simulink model "THEFINAL"  (R2020b)
settings: Solver=VariableStepAuto  StartTime=0.0  StopTime=60  RelTol=1e-3
values from neighbouring files (symbols this model uses):
  A_2 = zeros(3)    [Trial_Script.m]
  A_AD = horzcat(A_i, A_ii)    [Trial_Script.m]
  A_kal = [0 0 0 1 0 0 ... (first row only)    [Trial_Script.m]
  B_2 = I_inv    [Trial_Script.m]
  B_AD = horzcat(B_i, B_ii)    [Trial_Script.m]
  B_kal = [0 0 0 0 0 0 ... (first row only)    [Trial_Script.m]
  C_2 = eye(3)    [Trial_Script.m]
  C_AD = eye(6)    [Trial_Script.m]
  C_kal = eye(6)    [Trial_Script.m]
  D_2 = zeros(3)    [Trial_Script.m]
  D_AD = zeros(6)    [Trial_Script.m]
  D_kal = zeros(6)    [Trial_Script.m]
  f_prop = 100    [Trial_Script.m]
  Fb1_l = -100000    [Trial_Script.m]
  Fb1_u = 100000    [Trial_Script.m]
  Fb2_l = -100000    [Trial_Script.m]
  Fb2_u = 100000    [Trial_Script.m]
  Fb3_l = -100000    [Trial_Script.m]
  Fb3_u = 100000    [Trial_Script.m]
  Fb4_l = -100000    [Trial_Script.m]
  Fb4_u = 100000    [Trial_Script.m]
  Fc1_l = -30000    [Trial_Script.m]
  Fc1_u = 30000    [Trial_Script.m]
  Fc2_l = -30000    [Trial_Script.m]
  Fc2_u = 30000    [Trial_Script.m]
  Fc3_l = -30000    [Trial_Script.m]
  Fc3_u = 30000    [Trial_Script.m]
  Ft1_l = -100000    [Trial_Script.m]
  Ft1_u = 100000    [Trial_Script.m]
  Ft2_l = -100000    [Trial_Script.m]
  Ft2_u = 100000    [Trial_Script.m]
  Ft3_l = -100000    [Trial_Script.m]
  Ft3_u = 100000    [Trial_Script.m]
  Ft4_l = -100000    [Trial_Script.m]
  Ft4_u = 100000    [Trial_Script.m]
  g = 9.81    [Trial_Script.m]
  m = 645    [Trial_Script.m]    (also in testing_file.m = (abs(max(z)) + abs(min(z)))/(abs(max(y)) + abs(min(y))); wind_stuff.m = (abs(max(z)) + abs(min(z)))/(abs(max(y)) + abs(min(y))))
  r_0 = Tzy_Shard*[90; -125; 160]    [Trial_Script.m]
  rho = 1.225    [Trial_Script.m]
  T = 10.5    [Trial_Script.m]
  time_delay = 0.1    [Trial_Script.m]
  Tx_aero = [1 0 0 ... (first row only)    [Trial_Script.m]
  Tzy_Shard = [cos(pi/2) -sin(pi/2) 0; sin(pi/2) cos(pi/2) 0; 0 0 1]*[1 0 0 ... (first row only)    [Reading_Shard_Data.m]    (also in Trial_Script.m)
  Tzy_Shard_inv = inv(Tzy_Shard)    [Trial_Script.m]
  u_0 = a(1:d,1)    [Reading_Shard_Data.m]    (also in Trial_Script.m = a(1:d_shard,1); testing_file.m)
  u_1 = a(1:d,2)    [Reading_Shard_Data.m]    (also in Trial_Script.m = a(1:d_shard,2); testing_file.m)
  u_2 = a(1:d,3)    [Reading_Shard_Data.m]    (also in Trial_Script.m = a(1:d_shard,3); testing_file.m)
  v_0 = Tzy_Shard*V0_shard    [Trial_Script.m]
  w_0 = [0;0;0]    [Trial_Script.m]
  xdata = a(1:d_shard,4)    [Trial_Script.m]
  ydata = a(1:d_shard,5)    [Trial_Script.m]
  zdata = a(1:d_shard,6)    [Trial_Script.m]
  ZI_Cx = model_Cx(XI_Cx, YI_Cx)    [Trial_Script.m]
  ZI_Cy = model_Cy(XI_Cy, YI_Cy)    [Trial_Script.m]
  ZI_Cz = model_Cz(XI_Cz, YI_Cz)    [Trial_Script.m]
  ZI_p = model_p(XI_p, YI_p)    [Trial_Script.m]
  ZI_q = model_q(XI_q, YI_q)    [Trial_Script.m]
  ZI_r = model_r(XI_r, YI_r)    [Trial_Script.m]
undefined symbols (not defined in the file or in its folder): C_D, Continuous, S, Time
libraries: pid_lib x3, dspsigops x3, fuzblock x3, dspindex x3, ctrlSharedLib x2, simulink x1, mpclib x1, dspmathops x1, cstblocks x1
(part 2 of 2)

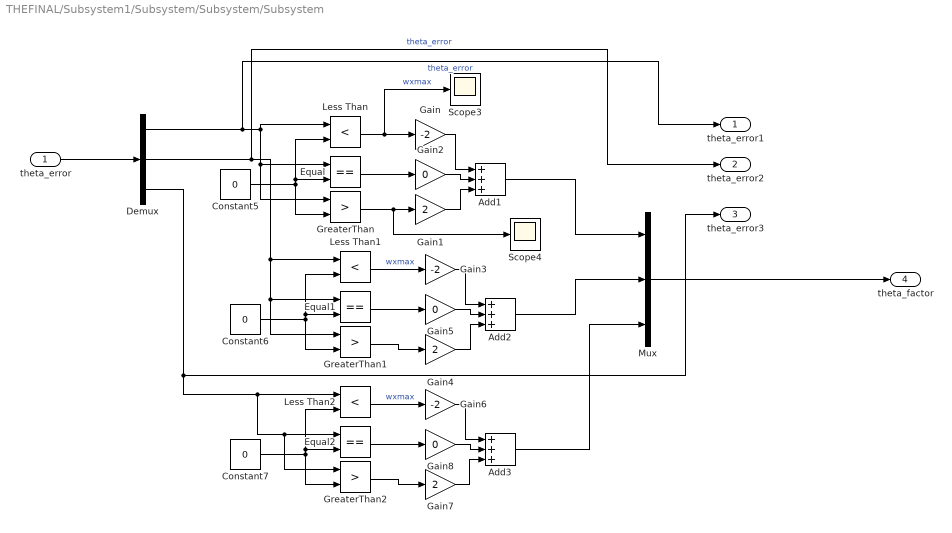
== system THEFINAL/Subsystem1/Subsystem/Subsystem/Subsystem ==
  theta_error : Inport
  Add1 : Sum  Inputs=+++
  Add2 : Sum  Inputs=+++
  Add3 : Sum  Inputs=+++
  Constant5 : Constant  Value=0
  Constant6 : Constant  Value=0
  Constant7 : Constant  Value=0
  Demux : Demux  Outputs=3
  Equal : RelationalOperator  Operator===  OutDataTypeStr=boolean  RndMeth=Simplest
  Equal1 : RelationalOperator  Operator===  OutDataTypeStr=boolean  RndMeth=Simplest
  Equal2 : RelationalOperator  Operator===  OutDataTypeStr=boolean  RndMeth=Simplest
  Gain : Gain  Gain=-2
  Gain1 : Gain  Gain=2
  Gain2 : Gain  Gain=0
  Gain3 : Gain  Gain=-2
  Gain4 : Gain  Gain=2
  Gain5 : Gain  Gain=0
  Gain6 : Gain  Gain=-2
  Gain7 : Gain  Gain=2
  Gain8 : Gain  Gain=0
  GreaterThan : RelationalOperator  Operator=>  OutDataTypeStr=boolean  RndMeth=Simplest
  GreaterThan1 : RelationalOperator  Operator=>  OutDataTypeStr=boolean  RndMeth=Simplest
  GreaterThan2 : RelationalOperator  Operator=>  OutDataTypeStr=boolean  RndMeth=Simplest
  Less Than : RelationalOperator  Operator=<  OutDataTypeStr=boolean  RndMeth=Simplest
  Less Than1 : RelationalOperator  Operator=<  OutDataTypeStr=boolean  RndMeth=Simplest
  Less Than2 : RelationalOperator  Operator=<  OutDataTypeStr=boolean  RndMeth=Simplest
  Mux : Mux  Inputs=3
  Scope3 : Scope
  Scope4 : Scope
  theta_error1 : Outport
  theta_error2 : Outport  Port=2
  theta_error3 : Outport  Port=3
  theta_factor : Outport  Port=4
  wires:
  Add1/1 -> Mux/1
  Constant5/1 -> Equal/2, Less Than/2, GreaterThan/2
  Equal2/1 -> Gain8/1
  Demux/1 -> theta_error1/1, GreaterThan/1, Equal/1, Less Than/1  "theta_error"
  GreaterThan2/1 -> Gain7/1
  Gain1/1 -> Add1/3
  Gain7/1 -> Add3/3
  Less Than1/1 -> Gain3/1  "wxmax"
  Gain6/1 -> Add3/1
  Equal/1 -> Gain2/1
  Gain5/1 -> Add2/2
  Add3/1 -> Mux/3
  GreaterThan/1 -> Scope4/1, Gain1/1
  Constant6/1 -> Equal1/2, Less Than1/2, GreaterThan1/2
  Demux/3 -> theta_error3/1, GreaterThan2/1, Equal2/1, Less Than2/1
  Gain3/1 -> Add2/1
  Constant7/1 -> Equal2/2, Less Than2/2, GreaterThan2/2
  Equal1/1 -> Gain5/1
  Gain8/1 -> Add3/2
  Gain4/1 -> Add2/3
  GreaterThan1/1 -> Gain4/1
  Gain/1 -> Add1/1
  Demux/2 -> theta_error2/1, GreaterThan1/1, Equal1/1, Less Than1/1  "theta_error"
  Gain2/1 -> Add1/2
  Add2/1 -> Mux/2
  Less Than/1 -> Scope3/1, Gain/1  "wxmax"
  Less Than2/1 -> Gain6/1  "wxmax"
  theta_error/1 -> Demux/1
  Mux/1 -> theta_factor/1

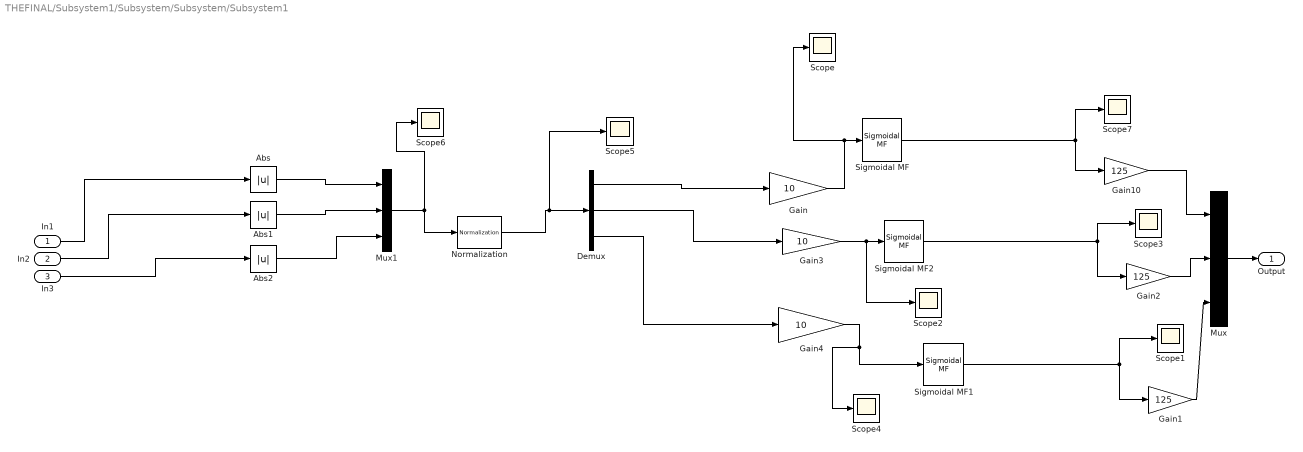
== system THEFINAL/Subsystem1/Subsystem/Subsystem/Subsystem1 ==
  In1 : Inport
  In2 : Inport  Port=2
  In3 : Inport  Port=3
  Abs : Abs
  Abs1 : Abs
  Abs2 : Abs
  Demux : Demux  Outputs=3
  Gain : Gain  Gain=10
  Gain1 : Gain  Gain=125
  Gain10 : Gain  Gain=125
  Gain2 : Gain  Gain=125
  Gain3 : Gain  Gain=10
  Gain4 : Gain  Gain=10
  Mux : Mux  Inputs=3
  Mux1 : Mux  Inputs=3
  Normalization : dspmathops/Normalization  NormType=Squared 2-norm  Bias=1e-10  NormOver=Each column  Dimension=1  roundingMode=Floor  overflowMode=off  accumDataTypeStr=Inherit: Same as product output  accumLastDataTypeStr=Inherit: Same as product output  outputDataTypeStr=Inherit: Same as product output  outputMin=[]  outputMax=[]  outputLastDataTypeStr=Inherit: Same as product output
  Scope{,1..7} (8 alike) : Scope
  Sigmoidal MF : fuzblock/Membership  Functions/Sigmoidal MF  a=10^(-8)  c=1000
      settings: SourceProductBaseCode=FL
  Sigmoidal MF1 : fuzblock/Membership  Functions/Sigmoidal MF  a=10^(-8)  c=1000
      settings: SourceProductBaseCode=FL
  Sigmoidal MF2 : fuzblock/Membership  Functions/Sigmoidal MF  a=10^(-8)  c=1000
      settings: SourceProductBaseCode=FL
  Output : Outport
  wires:
  Gain2/1 -> Mux/2
  Gain10/1 -> Mux/1
  Sigmoidal MF1/1 -> Gain1/1, Scope1/1
  Sigmoidal MF/1 -> Gain10/1, Scope7/1
  Sigmoidal MF2/1 -> Gain2/1, Scope3/1
  Gain/1 -> Scope/1, Sigmoidal MF/1
  Gain1/1 -> Mux/3
  Gain3/1 -> Scope2/1, Sigmoidal MF2/1
  In2/1 -> Abs1/1
  In1/1 -> Abs/1
  In3/1 -> Abs2/1
  Mux/1 -> Output/1
  Abs/1 -> Mux1/1
  Abs1/1 -> Mux1/2
  Gain4/1 -> Scope4/1, Sigmoidal MF1/1
  Abs2/1 -> Mux1/3
  Demux/3 -> Gain4/1
  Demux/1 -> Gain/1
  Demux/2 -> Gain3/1
  Mux1/1 -> Normalization/1, Scope6/1
  Normalization/1 -> Scope5/1, Demux/1

== matlab function THEFINAL/Transformation Subsystem/MATLAB Function2 ==
  data: theta_x input; Transformation_Mat output; theta_y input; theta_z input
function Transformation_Mat  = Euler(theta_x, theta_y, theta_z)

a = cos(theta_x)*cos(theta_z);
b = cos(theta_x)*sin(theta_z);
c = - sin(theta_x);
d = sin(theta_y)*sin(theta_x)*cos(theta_z) - cos(theta_y)*sin(theta_z);
e = sin(theta_y)*sin(theta_x)*sin(theta_z) + cos(theta_y)*cos(theta_z);
f = sin(theta_y)*cos(theta_x);
g = cos(theta_y)*sin(theta_x)*cos(theta_z) + sin(theta_y)*sin(theta_z);
h = cos(theta_y)*sin(theta_x)*sin(theta_z) - sin(theta_y)*cos(theta_z);
i = cos(theta_y)*cos(theta_x);

Transformation_Mat = [a b c;
    d e f;
    g h i];


end

== matlab function THEFINAL/GPS model/GPS Model ==
  settings: updateMethod=DISCRETE
  data: position input; newposition output
function newposition  = gps(position)

    % Input: position
    % Output: position with gps accuracies inclduded
    mu = 0; 
    sigma = 0.015;

    r1 = normrnd(mu, sigma);
    r2 = normrnd(mu, sigma);
    r3 = normrnd(mu, sigma);

    newposition = [0,0,0];

    newposition(1) = position(1) + r1;
    newposition(2) = position(2) + r2;
    newposition(3) = position(3) + r3;

end

== matlab function THEFINAL/Transformation Subsystem/MATLAB Function1 ==
  data: theta_x input; Transformation_Mat output; theta_y input; theta_z input
function Transformation_Mat  = Euler(theta_x, theta_y, theta_z)

a = cos(theta_x)*cos(theta_z);
b = cos(theta_x)*sin(theta_z);
c = - sin(theta_x);
d = sin(theta_y)*sin(theta_x)*cos(theta_z) - cos(theta_y)*sin(theta_z);
e = sin(theta_y)*sin(theta_x)*sin(theta_z) + cos(theta_y)*cos(theta_z);
f = sin(theta_y)*cos(theta_x);
g = cos(theta_y)*sin(theta_x)*cos(theta_z) + sin(theta_y)*sin(theta_z);
h = cos(theta_y)*sin(theta_x)*sin(theta_z) - sin(theta_y)*cos(theta_z);
i = cos(theta_y)*cos(theta_x);

Transformation_Mat = [a b c;
    d e f;
    g h i];


end

== matlab function THEFINAL/Propulsion commands module/Propeller firing function/MATLAB Function ==
  data: F_wanted input; F_c output; M_wanted input; F_t output; F_b output
function [F_c, F_t, F_b] = propeller_required_forces_control(F_wanted, M_wanted)

%% Load propeller arms data
xc_1 = 0.1;
yc_1 = 0;
zc_1 = 0.3;
xc_2 = 0.1;
yc_2 = 0;
zc_2 = 0.32;
xc_3 = 0.11;
yc_3 = 0;
zc_3 = 0.31;

xt_1 = 0.2;
yt_1 = 0.2;
zt_1 = 1;
xt_2 = 0.2;
yt_2 = 0.2;
zt_2 = 1;
xt_3 = 0.2;
yt_3 = 0.2;
zt_3 = 1;
xt_4 = 0.2;
yt_4 = 0.2;
zt_4 = 1;

xb_1 = 0.4;
yb_1 = 0.3;
zb_1 = 1.2;
xb_2 = 0.4;
yb_2 = 0.3;
zb_2 = 1.2;
xb_3 = 0.4;
yb_3 = 0.3;
zb_3 = 1.2;
xb_4 = 0.4;
yb_4 = 0.3;
zb_4 = 1.2;

%% Decompose force and moment input

F_x = F_wanted(1);
F_y = F_wanted(2);
F_z = F_wanted(3);

M_x = M_wanted(1);
M_y = M_wanted(2);
M_z = M_wanted(3);

%% Find control forces
A_control = [1 1 1;
    zc_1 -zc_2 -zc_3;
    -xc_1 -xc_2 xc_3];
A_cinv = inv(A_control);
force_control = [F_y; M_x; M_z];
controlvec = A_cinv*force_control;
F_c1 = controlvec(1);
F_c2 = controlvec(2);
F_c3 = controlvec(3);

%% Find top and bottom forces
A_tb = [-1 -1;
    2*(xt_1 + xb_1) -2*(xt_3 + xb_3)];
A_tbinv = inv(A_tb);
force_tb = [F_z; M_y];
tbvec = A_tbinv * force_tb;
f_front = tbvec(1);
F_t1 = f_front/4;
F_t2 = f_front/4;
F_b1 = f_front/4;
F_b2 = f_front/4;
f_back = tbvec(2);
F_t3 = f_back/4;
F_t4 = f_back/4;
F_b3 = f_back/4;
F_b4 = f_back/4;



%% Make matrix
F_c = [F_c1; F_c2; F_c3];
F_t = [F_t1; F_t2; F_t3; F_t4];
F_b = [F_b1; F_b2; F_b3; F_b4];
end

== matlab function THEFINAL/Subsystem2/MATLAB Function ==
  settings: updateMethod=DISCRETE
  data: angvel input; accelData output; acc input
function accelData = accelerometer(angvel, acc)

    %
    % Create gyroscope sensor object
    params = accelparams;
    
    % Parameters for simulated signal
    N = 1;       % Number of samples
    Fs = 100000;       % Sampling rate
    %Fc = 0.25;      % Sinusoidal frequency
    
    
    % Create arrays
    t = (0:(1/Fs):((N-1)/Fs)).';
    acc = acc;          %Input accelerations
    orient = quaternion.ones(N, 1);
    angvel = angvel;
    
    % Generate acceleration data
    imu = imuSensor('SampleRate', Fs, 'Accelerometer', params);
    imu.Accelerometer.MeasurementRange = 1000;   % Maximum acceleration accelerometer can measure
    imu.Accelerometer.Resolution = 1/Fs;           % Step size of digital measurements
    
    % Biases
    imu.Accelerometer.BiasInstability = 0.000000000001; 7.5 / 1000 * 9.81;
    imu.Accelerometer.NoiseDensity = 0.000000000001;%150 / 1000 / 1000 * 9.81 /10; 
    imu.Accelerometer.TemperatureBias = 50 / 1000 / 1000 * 9.81;
    
  
    
    accelData = imu(acc, angvel, orient);
    
    accelData(:,3) = accelData(:,3) - 9.81;

    accelData(:,1) = accelData(:,1) * -1;
    accelData(:,2) = accelData(:,2) * -1;
    accelData(:,3) = accelData(:,3) * -1;

end

== matlab function THEFINAL/Gyroscope Model/MATLAB Function ==
  settings: updateMethod=DISCRETE
  data: xvel input; yvel input; zvel input; gyroData output; acc input
function gyroData  = fungyroscope(xvel, yvel, zvel, acc)
   
    % Create gyroscope sensor object
    params = gyroparams;         
    
    % Parameters for simulated signal
    N = 1;       % Number of samples
    Fs = 100;       % Sampling rate
    Fc = 0.25;      % Sinusoidal frequency
    
    % Create arrays
    t = (0:(1/Fs):((N-1)/Fs)).';
    acc = acc;          % Input accelerations
    angvel = [xvel,yvel,zvel];
    %angvel(:,1) = 8*sin(2*pi*Fc*t);
    
    % Generate gyroscopic data
    imu = imuSensor('SampleRate', Fs, 'Gyroscope', params);
    imu.Gyroscope.MeasurementRange = 6.5;   % Maximum angular velocity gyroscope can measure
    imu.Gyroscope.Resolution = 1/Fs;           % Step size of digital measurements
    
    % Biases
    
    imu.Gyroscope.BiasInstability = 0.12 * 3.14159 / 180;       % rad/hr
    imu.Gyroscope.NoiseDensity = 0.15 * 3.14159 / 180;          % rad/s
    imu.Gyroscope.RandomWalk = 0.017 * 3.14159 / 180;           % rad/sqrt(hr)
    imu.Gyroscope.TemperatureBias = 0.25 * 3.14159 / 180;       % rad/s
    %imu.Gyroscope.AccelerationBias = 0.3;
    
    % Define real accelerations
    %acc(:,1) = 1;
    [~, gyroData] = imu(acc, angvel, eye(3));
    

end

== matlab function THEFINAL/Propulsion commands module/Subsystem3/MATLAB Function ==
  data: Fc input; Fx_acc output; Ft input; Fb input; Fy_acc output; Fz_acc output; Mx_acc output; My_acc output; Mz_acc output
function [Fx_acc,Fy_acc, Fz_acc, Mx_acc, My_acc, Mz_acc] = fcn(Fc, Ft, Fb)

%% Load propeller arms data
xc_1 = 0.1;
yc_1 = 0;
zc_1 = 0.3;
xc_2 = 0.1;
yc_2 = 0;
zc_2 = 0.32;
xc_3 = 0.11;
yc_3 = 0;
zc_3 = 0.31;

xt_1 = 0.2;
yt_1 = 0.2;
zt_1 = 1;
xt_2 = 0.2;
yt_2 = 0.2;
zt_2 = 1;
xt_3 = 0.2;
yt_3 = 0.2;
zt_3 = 1;
xt_4 = 0.2;
yt_4 = 0.2;
zt_4 = 1;

xb_1 = 0.4;
yb_1 = 0.3;
zb_1 = 1.2;
xb_2 = 0.4;
yb_2 = 0.3;
zb_2 = 1.2;
xb_3 = 0.4;
yb_3 = 0.3;
zb_3 = 1.2;
xb_4 = 0.4;
yb_4 = 0.3;
zb_4 = 1.2;


%% Split vectors
Fx_acc = 0;

A_control = [1 1 1;
    zc_1 -zc_2 -zc_3;
    -xc_1 -xc_2 xc_3];
ab_control = A_control*Fc;
Fy_acc = ab_control(1);
Mx_acc = ab_control(2);
Mz_acc = ab_control(3);

A_tb = [-1 -1;
    2*(xt_1 + xb_1) -2*(xt_3 + xb_3)];
F_front = Ft(1) + Ft(2) + Fb(1) + Fb(2);
F_back = Ft(3) + Ft(4) + Fb(3) + Fb(4);
Ftb_vec = [F_front; F_back];
Ab_tb = A_tb*Ftb_vec;

Fz_acc = Ab_tb(1);
My_acc = Ab_tb(2);

end

== matlab function THEFINAL/Subsystem4/MATLAB Function ==
  data: u_0 input; u_1 input; u_2 input; u0 output; xdata input; ydata input; zdata input; xpos input; ypos input; zpos input; u1 output; u2 output
function [u0, u1, u2] = wind_stuff(u_0, u_1, u_2, xdata, ydata, zdata, xpos, ypos, zpos)

x = xdata;
y = ydata;
z = zdata;

% z = m*y + c
x_p = xpos;
y_p = ypos;
z_p = zpos;
m = (abs(max(z)) + abs(min(z)))/(abs(max(y)) + abs(min(y)));
c = z(10) - m*y(10);
c_2 = z_p + m*y_p;
y_new = (c_2 - c)/(2*m);
z_new = m*y_new + c;

[~,~,idx]=unique(round(abs(z-z_new)),'stable');
minVal = z(idx==1);
z_val = minVal(1);
u0 = u_0(z_val);
u1 = u_1(z_val);
u2 = u_2(z_val);
end
